simulink library "LoadProfiles_lib"  (Simulink 8.1)
settings: Solver=ode45  StartTime=0.0  StopTime=10.0  RelTol=1e-3
settings Model: Creator=RE25624  LastModifiedBy=MGC4

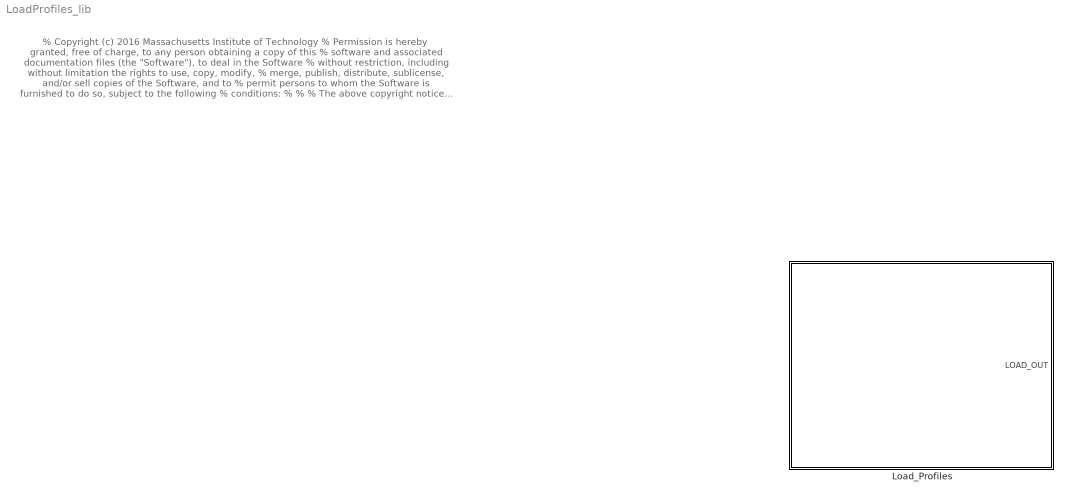
== system LoadProfiles_lib ==
  note: % Copyright (c) 2016 Massachusetts Institute of Technology
      | % Permission is hereby granted, free of charge, to any person obtaining a copy of this
      | % software and associated documentation files (the "Software"), to deal in the Software
      | % without restriction, including without limitation the rights to use, copy, modify,
      | % merge, publish, distribute, sublicense, and/or sell copies of the Software, and to
      | % permit persons to whom the Software is furnished to do so, subject to the following
      | % conditions:
      | %
      | %
      | % The above copyright notice and this permission notice shall be included in
      | % all copies or substantial portions of the Software.
      | %
      | % THE SOFTWARE IS PROVIDED "AS IS", WITHOUT WARRANTY OF ANY KIND, EXPRESS OR IMPLIED,
      | % INCLUDING BUT NOT LIMITED TO THE WARRANTIES OF MERCHANTABILITY, FITNESS FOR A
      | % PARTICULAR PURPOSE AND NONINFRINGEMENT. IN NO EVENT SHALL THE AUTHORS OR COPYRIGHT
      | % HOLDERS BE LIABLE FOR ANY CLAIM, DAMAGES OR OTHER LIABILITY, WHETHER IN AN ACTION
      | % OF CONTRACT, TORT OR OTHERWISE, ARISING FROM, OUT OF OR IN CONNECTION WITH THE
      | % SOFTWARE OR THE USE OR OTHER DEALINGS IN THE SOFTWARE.
      | %
      | %
      | %%
  Load_Profiles : Subsystem

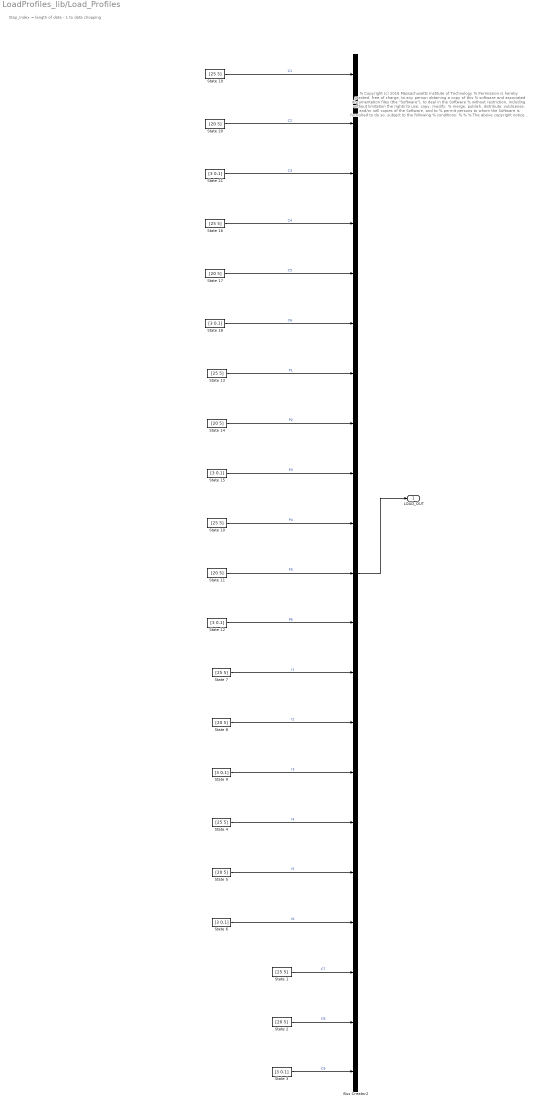
== system LoadProfiles_lib/Load_Profiles ==
  note: Stop_index = length of data - 1 to data chopping
  note: % Copyright (c) 2016 Massachusetts Institute of Technology
      | % Permission is hereby granted, free of charge, to any person obtaining a copy of this
      | % software and associated documentation files (the "Software"), to deal in the Software
      | % without restriction, including without limitation the rights to use, copy, modify,
      | % merge, publish, distribute, sublicense, and/or sell copies of the Software, and to
      | % permit persons to whom the Software is furnished to do so, subject to the following
      | % conditions:
      | %
      | %
      | % The above copyright notice and this permission notice shall be included in
      | % all copies or substantial portions of the Software.
      | %
      | % THE SOFTWARE IS PROVIDED "AS IS", WITHOUT WARRANTY OF ANY KIND, EXPRESS OR IMPLIED,
      | % INCLUDING BUT NOT LIMITED TO THE WARRANTIES OF MERCHANTABILITY, FITNESS FOR A
      | % PARTICULAR PURPOSE AND NONINFRINGEMENT. IN NO EVENT SHALL THE AUTHORS OR COPYRIGHT
      | % HOLDERS BE LIABLE FOR ANY CLAIM, DAMAGES OR OTHER LIABILITY, WHETHER IN AN ACTION
      | % OF CONTRACT, TORT OR OTHERWISE, ARISING FROM, OUT OF OR IN CONNECTION WITH THE
      | % SOFTWARE OR THE USE OR OTHER DEALINGS IN THE SOFTWARE.
      | %
      | %
      | %%
  Bus Creator2 : BusCreator  Inputs=21
  State {1,4,7,10,13,16,19} (7 alike) : Constant  Value=[25 5]
  State {2,5,8,11,14,17,20} (7 alike) : Constant  Value=[20 5]
  State {3,6,9,12,15,18,21} (7 alike) : Constant  Value=[3 0.1]
  LOAD_OUT : Outport
  wires:
  State 3/1 -> Bus Creator2/21  "C9"
  State 2/1 -> Bus Creator2/20  "C8"
  State 1/1 -> Bus Creator2/19  "C7"
  State 16/1 -> Bus Creator2/4  "C4"
  State 18/1 -> Bus Creator2/6  "C6"
  State 17/1 -> Bus Creator2/5  "C5"
  State 21/1 -> Bus Creator2/3  "C3"
  State 20/1 -> Bus Creator2/2  "C2"
  State 19/1 -> Bus Creator2/1  "C1"
  Bus Creator2/1 -> LOAD_OUT/1
  State 12/1 -> Bus Creator2/12  "P6"
  State 15/1 -> Bus Creator2/9  "P3"
  State 5/1 -> Bus Creator2/17  "I5"
  State 14/1 -> Bus Creator2/8  "P2"
  State 13/1 -> Bus Creator2/7  "P1"
  State 10/1 -> Bus Creator2/10  "P4"
  State 11/1 -> Bus Creator2/11  "P5"
  State 7/1 -> Bus Creator2/13  "I1"
  State 6/1 -> Bus Creator2/18  "I6"
  State 8/1 -> Bus Creator2/14  "I2"
  State 4/1 -> Bus Creator2/16  "I4"
  State 9/1 -> Bus Creator2/15  "I3"
